simulink model "stugverter_sil"  (R2026a)
settings: Solver=VariableStepAuto  StopTime=0.8  MaxStep=1e-5
PreLoadFcn:
  | if exist('init', 'file') ~= 2,   pDir = fileparts(fileparts(which(bdroot)));   if isempty(pDir), pDir = pwd; end;   addpath(fullfile(pDir, 'scripts'));   addpath(fullfile(pDir, 'models'));   addpath(pDir); end; init;
InitFcn:
  | if exist('init', 'file') ~= 2,   pDir = fileparts(fileparts(which(bdroot)));   if isempty(pDir), pDir = pwd; end;   addpath(fullfile(pDir, 'scripts'));   addpath(fullfile(pDir, 'models'));   addpath(pDir); end; init;
undefined symbols (not defined in the file): foc, sensor
settings Model: Creator=niklasprobst  LastModifiedBy=probst
settings DebuggingCC: ParameterPrecisionLossMsg=none

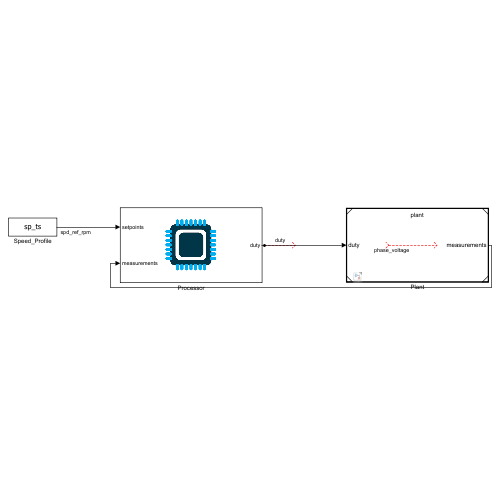
[thumbnail: Simulink's stored preview of the top-level diagram]
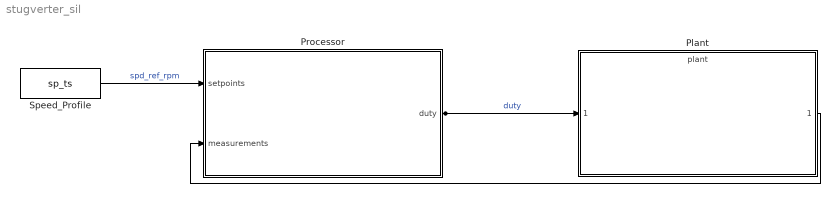
== system stugverter_sil ==
  Plant : ModelReference  ModelNameDialog=plant  SimulationMode=Normal  ModelReferenceVersion=1.2
  Processor : Subsystem
      settings: OpenFcn=open_system(gcb, 'force');
  Speed_Profile : FromWorkspace  VariableName=sp_ts
  wires:
  Speed_Profile/1 -> Processor/1(setpoints)  "spd_ref_rpm"
  Processor/1(duty) -> Plant/1  "duty"
  ? -> ?  "phase_voltage"
  Plant/1 -> Processor/2(measurements)

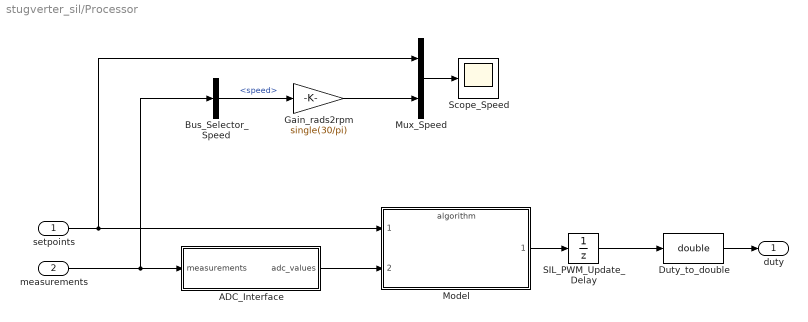
== system stugverter_sil/Processor ==
  setpoints : Inport  OutDataTypeStr=single
  measurements : Inport  Port=2  OutDataTypeStr=Bus: plant_measurement
  ADC_Interface : Subsystem
  Bus_Selector_Speed : BusSelector  OutputSignals=speed
  Duty_to_double : DataTypeConversion  OutDataTypeStr=double  SaturateOnIntegerOverflow=off  RndMeth=Floor
  Gain_rads2rpm : Gain  Gain=single(30/pi)  OutDataTypeStr=single
  Model : ModelReference  ModelNameDialog=algorithm  SimulationMode=Normal  ModelReferenceVersion=1.31
  Mux_Speed : Mux  Inputs=2
  SIL_PWM_Update_Delay : UnitDelay  InitialCondition=[0.5 0.5 0.5]  SampleTime=foc.Ts  StateName=sil_pwm_delay_state
  Scope_Speed : Scope
      settings: ActiveDisplayYMinimum=-579.96374511718739  ActiveDisplayYMaximum=5219.6737060546875  DataLoggingVariableName=scope_speed
  duty : Outport
  wires:
  setpoints/1 -> Model/1, Mux_Speed/1
  measurements/1 -> Bus_Selector_Speed/1, ADC_Interface/1(measurements)
  ADC_Interface/1(adc_values) -> Model/2
  Model/1 -> SIL_PWM_Update_Delay/1
  SIL_PWM_Update_Delay/1 -> Duty_to_double/1
  Duty_to_double/1 -> duty/1
  Bus_Selector_Speed/1 -> Gain_rads2rpm/1  "<speed>"
  Gain_rads2rpm/1 -> Mux_Speed/2
  Mux_Speed/1 -> Scope_Speed/1

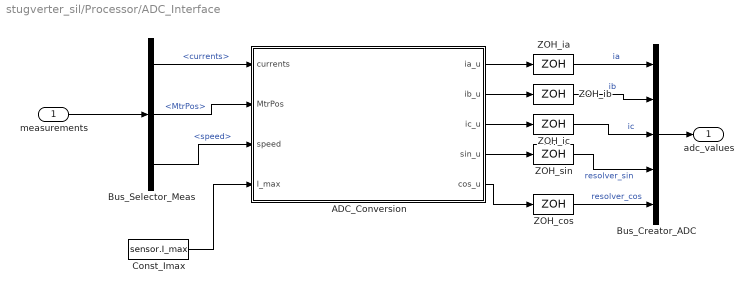
== system stugverter_sil/Processor/ADC_Interface ==
  measurements : Inport  OutDataTypeStr=Bus: plant_measurement
  ADC_Conversion : MATLAB Function  TreatAsAtomicUnit=on
  Bus_Creator_ADC : BusCreator  Inputs=5  OutDataTypeStr=Bus: adc_values  NonVirtualBus=on
  Bus_Selector_Meas : BusSelector  OutputSignals=currents,MtrPos,speed
  Const_Imax : Constant  Value=sensor.I_max
  ZOH_cos : ZeroOrderHold  SampleTime=foc.Ts
  ZOH_ia : ZeroOrderHold  SampleTime=foc.Ts
  ZOH_ib : ZeroOrderHold  SampleTime=foc.Ts
  ZOH_ic : ZeroOrderHold  SampleTime=foc.Ts
  ZOH_sin : ZeroOrderHold  SampleTime=foc.Ts
  adc_values : Outport  OutDataTypeStr=Bus: adc_values
  wires:
  measurements/1 -> Bus_Selector_Meas/1
  Bus_Selector_Meas/1 -> ADC_Conversion/1(currents)  "<currents>"
  Bus_Selector_Meas/2 -> ADC_Conversion/2(MtrPos)  "<MtrPos>"
  ADC_Conversion/1(ia_u) -> ZOH_ia/1
  ZOH_ia/1 -> Bus_Creator_ADC/1  "ia"
  ADC_Conversion/2(ib_u) -> ZOH_ib/1
  ZOH_ib/1 -> Bus_Creator_ADC/2  "ib"
  ADC_Conversion/3(ic_u) -> ZOH_ic/1
  ZOH_ic/1 -> Bus_Creator_ADC/3  "ic"
  ADC_Conversion/4(sin_u) -> ZOH_sin/1
  ZOH_sin/1 -> Bus_Creator_ADC/4  "resolver_sin"
  ADC_Conversion/5(cos_u) -> ZOH_cos/1
  ZOH_cos/1 -> Bus_Creator_ADC/5  "resolver_cos"
  Bus_Creator_ADC/1 -> adc_values/1
  Bus_Selector_Meas/3 -> ADC_Conversion/3(speed)  "<speed>"
  Const_Imax/1 -> ADC_Conversion/4(I_max)

== matlab function stugverter_sil/Processor/ADC_Interface/ADC_Conversion ==
  settings: updateMethod=DISCRETE  sampleTime=foc.Ts
  data: currents input; ia_u output; MtrPos input; speed input; I_max input; ib_u output; ic_u output; sin_u output; cos_u output
function [ia_u, ib_u, ic_u, sin_u, cos_u] = fcn(currents, MtrPos, speed, I_max)
% Infineon AURIX TC387 12-bit EVADC (0..4095, midpoint 2048)
scale_I = 2047 / I_max;
ia_c = round(2048 + currents(1) * scale_I);
ib_c = round(2048 + currents(2) * scale_I);
ic_c = round(2048 + currents(3) * scale_I);
ia_u = uint16(max(0, min(4095, ia_c)));
ib_u = uint16(max(0, min(4095, ib_c)));
ic_u = uint16(max(0, min(4095, ic_c)));

% 1.5-sample PWM + transport delay compensation
pos_comp = MtrPos + 1.5 * speed * 0.00005;
sin_c = round(2048 + sin(pos_comp) * 2047);
cos_c = round(2048 + cos(pos_comp) * 2047);
sin_u = uint16(max(0, min(4095, sin_c)));
cos_u = uint16(max(0, min(4095, cos_c)));
